simulink model "ExampleModel"  (R2016a)
settings: Solver=VariableStepAuto  StartTime=0.0  StopTime=10.0  RelTol=1e-3
undefined symbols (not defined in the file or in its folder): MP
libraries: library_mtu_simulink x2, simulink x1
settings Model: Creator=danielhaeufle  LastModifiedBy=danielhaeufle

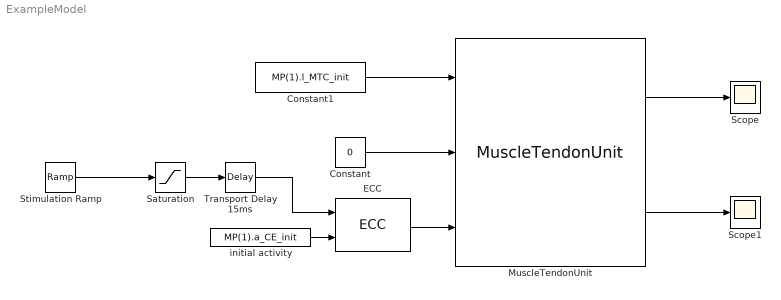
== system ExampleModel ==
  Constant : Constant  Value=0
  Constant1 : Constant  Value=MP(1).l_MTC_init
  ECC : library_mtu_simulink/ECC
  MuscleTendonUnit : library_mtu_simulink/MuscleTendonUnit  Mus_Param=MP(1)
  Saturation : Saturate  UpperLimit=1  LowerLimit=0.001
  Scope : Scope
  Scope1 : Scope
  Stimulation Ramp : simulink/Sources/Ramp  slope=0.1  start=0  X0=0
  Transport Delay 15ms : TransportDelay  DelayTime=0.015  InitialOutput=MP(1).a_CE_init
  initial activity : Constant  Value=MP(1).a_CE_init
  wires:
  Saturation/1 -> Transport Delay 15ms/1
  ECC/1 -> MuscleTendonUnit/3
  Transport Delay 15ms/1 -> ECC/1
  initial activity/1 -> ECC/2
  Stimulation Ramp/1 -> Saturation/1
  Constant/1 -> MuscleTendonUnit/2
  Constant1/1 -> MuscleTendonUnit/1
  MuscleTendonUnit/1 -> Scope/1
  MuscleTendonUnit/2 -> Scope1/1
